simulink model "Task2_1_Robust_CLF"  (R2024b)
settings: Solver=ode45  StartTime=0.0  StopTime=30  MaxStep=0.01  RelTol=1e-3
InitFcn:
  | if ~exist('params','var'), params=System_Parameters(); end; if ~exist('simcfg','var'), simcfg=Simulink_Config(params); end;
undefined symbols (not defined in the file): params, simcfg
settings Model: Creator=LAPTOPASADI  LastModifiedBy=LAPTOPASADI

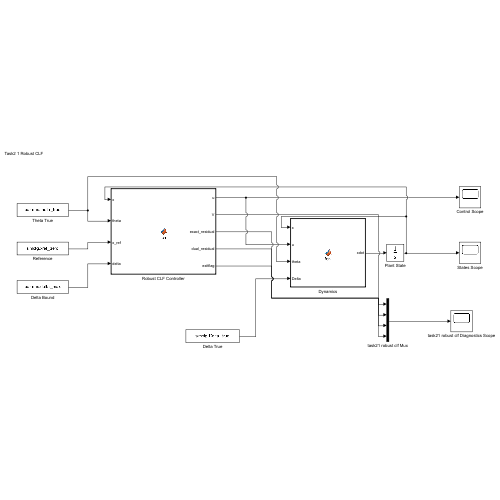
[thumbnail: Simulink's stored preview of the top-level diagram]
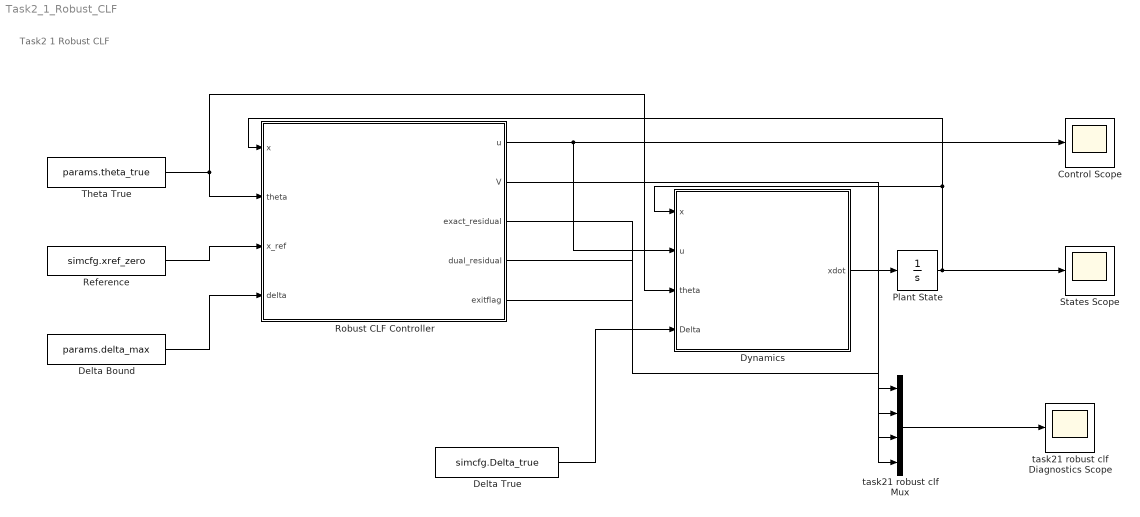
== system Task2_1_Robust_CLF ==
  note: Task2 1 Robust CLF
  Control Scope : Scope
  Delta Bound : Constant  Value=params.delta_max
  Delta True : Constant  Value=simcfg.Delta_true
  Dynamics : MATLAB Function  TreatAsAtomicUnit=on
  Plant State : Integrator  InitialCondition=simcfg.x0_task11
  Reference : Constant  Value=simcfg.xref_zero
  Robust CLF Controller : MATLAB Function  TreatAsAtomicUnit=on
  States Scope : Scope
  Theta True : Constant  Value=params.theta_true
  task21 robust clf Diagnostics Scope : Scope
  task21 robust clf Mux : Mux
  wires:
  Plant State/1 -> Robust CLF Controller/1(x), Dynamics/1(x), States Scope/1
  Theta True/1 -> Robust CLF Controller/2(theta), Dynamics/3(theta)
  Reference/1 -> Robust CLF Controller/3(x_ref)
  Delta Bound/1 -> Robust CLF Controller/4(delta)
  Robust CLF Controller/1(u) -> Control Scope/1, Dynamics/2(u)
  Delta True/1 -> Dynamics/4(Delta)
  Dynamics/1(xdot) -> Plant State/1
  Robust CLF Controller/2(V) -> task21 robust clf Mux/1
  Robust CLF Controller/3(exact_residual) -> task21 robust clf Mux/2
  Robust CLF Controller/4(dual_residual) -> task21 robust clf Mux/3
  Robust CLF Controller/5(exitflag) -> task21 robust clf Mux/4
  task21 robust clf Mux/1 -> task21 robust clf Diagnostics Scope/1

== matlab function Task2_1_Robust_CLF/Dynamics ==
  data: x input; u input; xdot output; theta input; Delta input
function xdot = fcn(x,u,theta,Delta)
G = [0 0 40.75371832714017 8.6858779355964231;0 5.9859154929577469 0 0;0 0 2.4098880670272087 -9.893830239002293];
x=reshape(x,6,1);
u=reshape(u,4,1);
theta=reshape(theta,6,1);
Delta=reshape(Delta,4,4);

phi = x(1);
pitch = x(2);
p = x(4);
q = x(5);
r = x(6);

cphi = cos(phi);
sphi = sin(phi);
cpitch = cos(pitch);
if abs(cpitch) < 1e-6
    cpitch = sign(cpitch+eps)*1e-6;
end
tpitch = sin(pitch)/cpitch;

J = [1, sphi*tpitch, cphi*tpitch;
     0, cphi,         -sphi;
     0, sphi/cpitch,  cphi/cpitch];
f0 = [J*[p;q;r]; zeros(3,1)];
Fomega = [p*q, -q*r, 0, 0, 0, -p;
          0, 0, p*r, -(p^2-r^2), 0, -q;
          -q*r, 0, 0, 0, p*q, -r];
F = [zeros(3,6); Fomega];
g = [zeros(3,4); G];
xdot = f0+F*theta+g*(eye(4)+Delta)*u;
end

== matlab function Task2_1_Robust_CLF/Robust CLF Controller ==
  data: x input; u output; theta input; x_ref input; delta input; V output; exact_residual output; dual_residual output; exitflag output
function [u,V,exact_residual,dual_residual,exitflag] = fcn(x,theta,x_ref,delta)
P=[0.11250000000000002 0 0 0.012500000000000001 0 0;0 0.11250000000000002 0 0 0.012500000000000001 0;0 0 0.11250000000000002 0 0 0.012500000000000001;0.012500000000000001 0 0 0.015625 0 0;0 0.012500000000000001 0 0 0.015625 0;0 0 0.012500000000000001 0 0 0.015625]; G=[0 0 40.75371832714017 8.6858779355964231;0 5.9859154929577469 0 0;0 0 2.4098880670272087 -9.893830239002293]; gamma=0.5;
x=reshape(x,6,1);theta=reshape(theta,6,1);x_ref=reshape(x_ref,6,1);
lower=[-inf;-inf;-inf;-inf]; upper=[inf;inf;inf;inf];
[V,omega,phiV,a]=clf_terms(x,x_ref,P,G);
drift=omega+phiV'*theta;
b=-gamma*V-drift;
beta=delta*norm(a,2);
[u,exitflag]=solve_l1(a,b,beta,lower,upper);
if exitflag<=0
    [u,exitflag]=solve_spectral(a,b,beta,lower,upper);
end
dual_residual=drift+a*u+beta*sum(abs(u))+gamma*V;
exact_residual=drift+a*u+beta*norm(u,2)+gamma*V;
end

function [V,omega,phiV,LgV]=clf_terms(x,x_ref,P,G)
phi=x(1); pitch=x(2); w=x(4:6);
[J,Jphi,Jpitch]=kinematics(phi,pitch);
rates=J*w; Jdot=Jphi*rates(1)+Jpitch*rates(2);
eta=[x(1:3)-x_ref(1:3);rates];
p=x(4);q=x(5);r=x(6);
Fw=[p*q,-q*r,0,0,0,-p;0,0,p*r,-(p^2-r^2),0,-q;-q*r,0,0,0,p*q,-r];
grad=2*P*eta; V=eta'*P*eta;
omega=grad(1:3)'*rates+grad(4:6)'*(Jdot*w);
phiV=(J*Fw)'*grad(4:6); LgV=grad(4:6)'*(J*G);
end

function [J,Jphi,Jpitch]=kinematics(phi,pitch)
c=cos(phi);s=sin(phi);cp=cos(pitch);
if abs(cp)<1e-6,cp=sign(cp+eps)*1e-6;end
t=sin(pitch)/cp;sec=1/cp;
J=[1,s*t,c*t;0,c,-s;0,s*sec,c*sec];
Jphi=[0,c*t,-s*t;0,-s,-c;0,c*sec,-s*sec];
Jpitch=[0,s*sec^2,c*sec^2;0,0,0;0,s*sec*t,c*sec*t];
end

function [best,flag]=solve_l1(a,b,beta,lower,upper)
tol=1e-10; best=zeros(4,1); best_cost=inf; flag=-2;
unbounded=all(isinf(lower)&lower<0)&&all(isinf(upper)&upper>0);
for mask=0:15
    signs=zeros(4,1);
    for j=1:4
        if bitget(mask,j),signs(j)=1;else,signs(j)=-1;end
    end
    lo=lower;hi=upper;positive=signs>0;
    lo(positive)=max(lo(positive),0);hi(~positive)=min(hi(~positive),0);
    if any(lo>hi),continue;end
    row=a+beta*signs';
    if unbounded
        if b>=-tol
            candidate=zeros(4,1);ok=1;
        else
            direction=-row';direction(signs.*direction<0)=0;
            denominator=row*direction;
            if denominator<-eps,candidate=(b/denominator)*direction;ok=1;
            else,candidate=zeros(4,1);ok=-2;end
        end
    else
        [candidate,ok]=project_origin(row,b,lo,hi,tol);
    end
    if ok>0 && a*candidate+beta*sum(abs(candidate))<=b+tol
        cost=candidate'*candidate;
        if cost<best_cost,best=candidate;best_cost=cost;flag=1;end
    end
end
end

function [u,flag]=project_origin(a,b,lower,upper,tol)
u=min(max(zeros(4,1),lower),upper);
if a*u<=b+tol,flag=1;return;end
umin=u;umin(a>0)=lower(a>0);umin(a<0)=upper(a<0);
if a*umin>b+tol,u=umin;flag=-2;return;end
lo=0;hi=1;
while a*min(max(-hi*a',lower),upper)>b
    hi=2*hi;if hi>1e12,u=umin;flag=-2;return;end
end
for k=1:80
    mid=0.5*(lo+hi);candidate=min(max(-mid*a',lower),upper);
    if a*candidate>b,lo=mid;else,hi=mid;end
end
u=min(max(-hi*a',lower),upper);flag=1;
end

function [u,flag]=solve_spectral(a,b,beta,lower,upper)
tol=1e-10;u=min(max(zeros(4,1),lower),upper);
if a*u+beta*norm(u)<=b+tol,flag=1;return;end
lo=0;hi=1;previous=nan(4,1);
while true
    candidate=min(max(-hi*a',lower),upper);
    if a*candidate+beta*norm(candidate)<=b+tol,break;end
    if all(isfinite(previous))&&norm(candidate-previous,inf)<=eps,u=candidate;flag=-2;return;end
    previous=candidate;hi=2*hi;
    if hi>1e12,u=candidate;flag=-2;return;end
end
for k=1:80
    mid=0.5*(lo+hi);candidate=min(max(-mid*a',lower),upper);
    if a*candidate+beta*norm(candidate)>b,lo=mid;else,hi=mid;end
end
u=min(max(-hi*a',lower),upper);flag=1;
end
